simulink model "Main_Firmware"  (R2024b)
settings: Solver=FixedStepDiscrete  StartTime=0.0  StopTime=Inf  FixedStep=5e-06  RelTol=1e-3
values from neighbouring files (symbols this model uses):
  A_f = 1.24    [Minh_Inverter_Init.m]
  C_d = 0.7041    [Minh_Inverter_Init.m]
  C_rr = 0.02    [Minh_Inverter_Init.m]
  Current_max = min(InvCurr,mCurr)    [Minh_Inverter_Init.m]
  Encoder_Offset = -17.439*pi/180    (= -0.304367968255)    [Minh_Inverter_Init.m]
  EPWM_F = 200000    [Minh_Inverter_Init.m]
  g = 9.8    [Minh_Inverter_Init.m]
  J = mrot*r^2/k^2 + 0.0045    (= 0.8303048)    [Minh_Inverter_Init.m]
  k = 1    [Minh_Inverter_Init.m]
  lambda = 0.0375    [Minh_Inverter_Init.m]
  Ld = 0.1e-3    (= 0.0001)    [Minh_Inverter_Init.m]
  Lq = Ld    (= 0.0001)    [Minh_Inverter_Init.m]
  m = 1    [Minh_Inverter_Init.m]
  ppair = 4    [Minh_Inverter_Init.m]
  r = 0.4064/2    (= 0.2032)    [Minh_Inverter_Init.m]
  rho = 1.2    [Minh_Inverter_Init.m]
  Rs = (Rpp^2)/(Rpp*3)    (= 0.00433333333333)    [Minh_Inverter_Init.m]
  speed_max = rpm_max*2*pi/60    (= 523.598775598)    [Minh_Inverter_Init.m]
  Torque_max = Current_max*3*lambda*ppair/2    [Minh_Inverter_Init.m]
  Voltage_max = min(V_bat,mVolt)    [Minh_Inverter_Init.m]
undefined symbols (not defined in the file or in its folder): DiscIntNeverNeededParam, dspblkCoreblockFVToolHelper, gcbh, GPTRIP1SEL, TZ1
libraries: c2802xlib x4, c28004xlib x3, slpidlib x3, simulink x2, spsabctodq0Lib x2, spsdq0toabcLib x1
settings Model: SimulationMode=external  ExtModeTrigDuration=8  Creator=minhp  LastModifiedBy=minhp
settings OptimizationCC: DefaultUnderspecifiedDataType=single  EnhancedBackFolding=on  PassReuseOutputArgsAs=Individual arguments  MaxStackSize=1024  OptimizeBlockOrder=speed  DifferentSizesBufferReuse=on  OptimizationCustomize=off  EfficientTunableParamExpr=on
settings DebuggingCC: SingleTaskRateTransMsg=warning  ParameterTunabilityLossMsg=error
settings HardwareCC: ProdBitPerChar=16  ProdBitPerInt=16  ProdBitPerPointer=32  ProdBitPerSizeT=32  ProdBitPerPtrDiffT=32  ProdLargestAtomicInteger=Integer  ProdLargestAtomicFloat=None  ProdWordSize=16  ProdLongLongMode=on  ProdHWDeviceType=Texas Instruments->C2000  HardwareBoardFeatureSet=SoCBlockset
settings SFSimCC: MATLABDynamicMemAlloc=off
settings RTWCC: Description=Embedded Coder  SystemTargetFile=ert.tlc  HardwareBoard=TI Piccolo F280049C LaunchPad  TemplateMakefile=ert_default_tmf  Toolchain=Texas Instruments Code Composer Studio (C2000)  CodeProfilingSaveOptions=MetricsOnly
settings CodeAppCC: ForceParamTrailComments=on  IgnoreCustomStorageClasses=off  OperatorAnnotations=on  SimulinkDataObjDesc=on  SFDataObjDesc=on  InsertBlockDesc=on
settings ERTTargetCC: CodeReplacementLibrary=TI C28x  ExtModeTransport=4  ExtModeStaticAlloc=on  ExtModeAutomaticAllocSize=off  ExtModeStaticAllocSize=5000  ExtModeMexFile=ext_xcp  ExtModeIntrfLevel=Level2 - Open  InlinedParameterPlacement=Hierarchical  DynamicArrayContainerType=coder::array

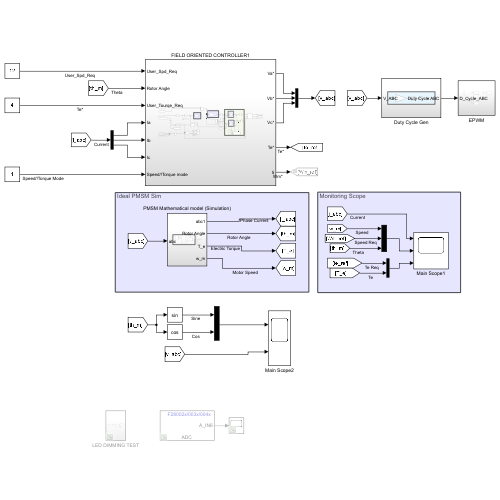
[thumbnail: Simulink's stored preview of the top-level diagram]
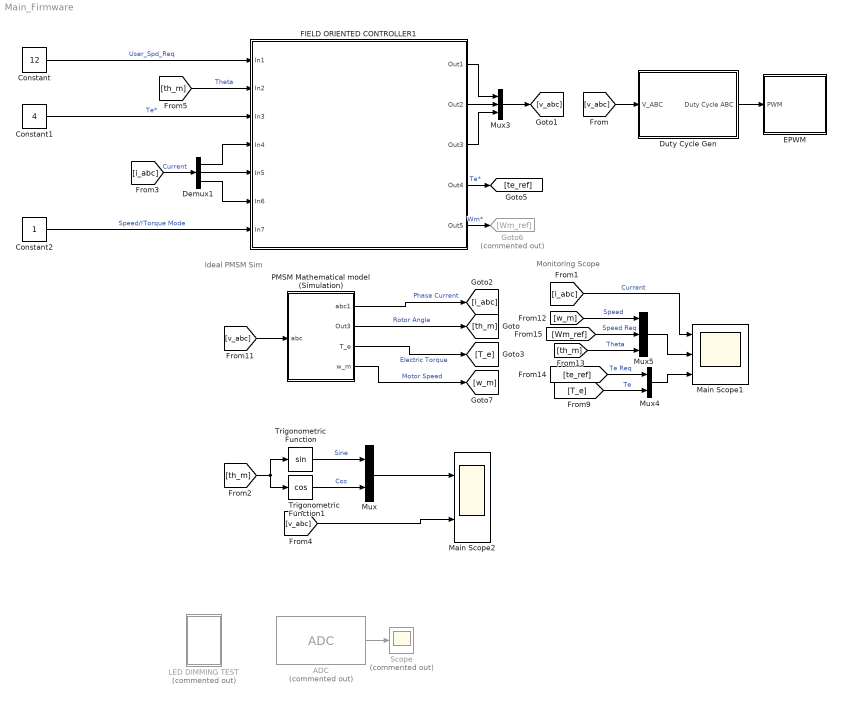
== system Main_Firmware ==
  note: Ideal PMSM Sim
  note: Monitoring Scope
  ADC : c2802xlib/ADC  Commented=on  blkParamProc=C2000_Type5  ADCModule=A  samplingMode=Single sample mode  ADCResolution=12-bit (Single-ended input)  useSOC1=SOC0  useSOC2=SOC0_SOC1  SOCAcquisitionWindow=8  SOCTriggerSource=Software  SOCInterruptTrigger=No ADCINT  Ts=0.001  dType=single  postInterrupt=off  interruptSel=ADCINT1  ADCINTContinuous=on  endma=off  chdma=1  conv1=ADCINA0  conv2=ADCINA0 and ADCINB0  conv1_Type4=ADCIN6  conv2_Type4=ADCIN0 and ADCIN1
      settings: LibrarySourceBlock=c28004xlib/ADC
  Constant : Constant  Value=12
  Constant1 : Constant  Value=4
  Constant2 : Constant
  Demux1 : Demux  Outputs=3
  Duty Cycle Gen : Subsystem
  EPWM : Subsystem
  FIELD ORIENTED CONTROLLER1 : Subsystem
  Goto6 : Goto  Commented=on  GotoTag=Wm_ref
  LED DIMMING TEST : Subsystem  Commented=on
  Main Scope1 : Scope  NumInputPorts=3
  Main Scope2 : Scope  NumInputPorts=2
  Mux : Mux  Inputs=2
  Mux3 : Mux  Inputs=3
  Mux4 : Mux  Inputs=2
  Mux5 : Mux  Inputs=3
  PMSM Mathematical model (Simulation) : Subsystem
  Scope : Scope  Commented=on
  Trigonometric Function : Trigonometry
  Trigonometric Function1 : Trigonometry  Operator=cos
  wires:
  ADC/1 -> Scope/1
  Duty Cycle Gen/1(Duty Cycle ABC) -> EPWM/1(PWM)
  PMSM Mathematical model (Simulation)/2(Out3) -> [th_m]  "Rotor Angle"
  PMSM Mathematical model (Simulation)/4(w_m) -> [w_m]  "Motor Speed"
  [v_abc] -> PMSM Mathematical model (Simulation)/1(abc)
  PMSM Mathematical model (Simulation)/1(abc1) -> [i_abc]  "Phase Current"
  PMSM Mathematical model (Simulation)/3(T_e) -> [T_e]  "Electric Torque"
  Constant1/1 -> FIELD ORIENTED CONTROLLER1/3(In3)  "Te*"
  FIELD ORIENTED CONTROLLER1/1(Out1) -> Mux3/1
  FIELD ORIENTED CONTROLLER1/4(Out4) -> [te_ref]  "Te*"
  FIELD ORIENTED CONTROLLER1/2(Out2) -> Mux3/2
  Mux3/1 -> [v_abc]
  FIELD ORIENTED CONTROLLER1/3(Out3) -> Mux3/3
  [i_abc] -> Demux1/1  "Current"
  [th_m] -> FIELD ORIENTED CONTROLLER1/2(In2)  "Theta"
  Demux1/2 -> FIELD ORIENTED CONTROLLER1/5(In5)
  Demux1/3 -> FIELD ORIENTED CONTROLLER1/6(In6)
  Constant2/1 -> FIELD ORIENTED CONTROLLER1/7(In7)  "Speed/!Torque Mode"
  Demux1/1 -> FIELD ORIENTED CONTROLLER1/4(In4)
  Constant/1 -> FIELD ORIENTED CONTROLLER1/1(In1)  "User_Spd_Req"
  FIELD ORIENTED CONTROLLER1/5(Out5) -> Goto6/1  "Wm*"
  [v_abc] -> Duty Cycle Gen/1(V_ABC)
  [th_m] -> Mux5/3  "Theta"
  [te_ref] -> Mux4/1  "Te Req"
  [T_e] -> Mux4/2  "Te"
  Mux5/1 -> Main Scope1/2
  [w_m] -> Mux5/1  "Speed"
  [Wm_ref] -> Mux5/2  "Speed Req"
  [i_abc] -> Main Scope1/1  "Current"
  Mux4/1 -> Main Scope1/3
  [th_m] -> Trigonometric Function1/1, Trigonometric Function/1
  Trigonometric Function1/1 -> Mux/2  "Cos"
  [v_abc] -> Main Scope2/2
  Trigonometric Function/1 -> Mux/1  "Sine"
  Mux/1 -> Main Scope2/1

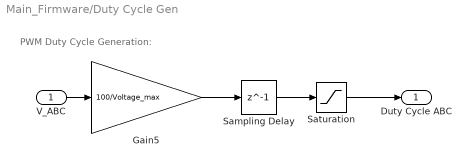
== system Main_Firmware/Duty Cycle Gen ==
  note: PWM Duty Cycle Generation:
  V_ABC : Inport
  Gain5 : Gain  Gain=100/Voltage_max
  Sampling Delay : Delay  DelayLength=1
  Saturation : Saturate  UpperLimit=100  LowerLimit=0
  Duty Cycle ABC : Outport
  wires:
  Sampling Delay/1 -> Saturation/1
  Gain5/1 -> Sampling Delay/1
  Saturation/1 -> Duty Cycle ABC/1
  V_ABC/1 -> Gain5/1

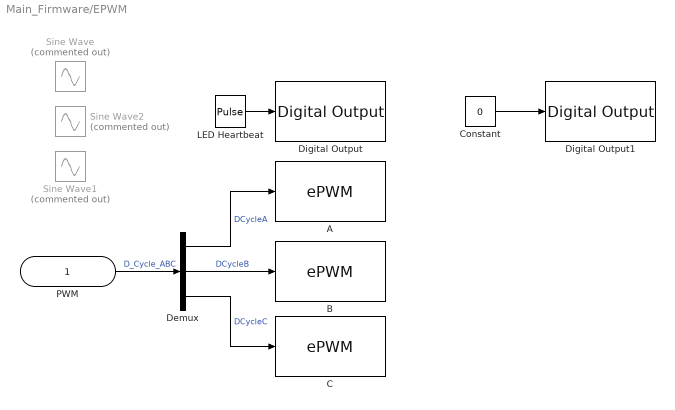
== system Main_Firmware/EPWM ==
  PWM : Inport
  A : c2802xlib/ePWM  PwmType=C2000_Type4  useModule=ePWM1  ePWMxLINKTBPRD=Not Linked  periodUnits=Seconds  timerSource=Specify via dialog  timerPeriod_clk=1/EPWM_F  timerPeriod_sec=1/EPWM_F  tbshadow=Counter equals to zero  countingMode=Up  phaseActiveEnable=Disable  phaseDirection=Count down after sync  phaseActive=0  synchronizationEnable=off  dcaevt1Sync=off  dcbevt1Sync=off  synchronizationOption=Disable  dcbevt1SyncOut=off  dcaevt1SyncOut=off  cmpdSyncOut=off  cmpcSyncOut=off  cmpbSyncOut=off  zeroSyncOut=off  swfSyncOut=off  perSynchronizationOption=Counter equals to period (CTR=PRD)  clockPrescale=1  HSclockPrescale=1  enswap=off  ePWMxAStatus=on  ePWMxAactionLogic1=Set  ePWMxAactionLogic2=Clear  ePWMxAactionLogic3=Clear  ePWMxAactionLogic4=Set  ePWMxAactionLogic5=Do nothing  ePWMxAactionLogic6=Do nothing  ePWMxACSFenable=off  ePWMxACSFvalue=Forcing disable  ePWMxASFreload=Zero  ePWMxBStatus=on  ePWMxBactionLogic1=Set  ePWMxBactionLogic2=Clear  ePWMxBactionLogic3=Clear  ePWMxBactionLogic4=Do nothing  ePWMxBactionLogic5=Do nothing  ePWMxBactionLogic6=Set  ePWMxBCSFenable=off  ePWMxBCSFvalue=Forcing disable  ePWMxBSFreload=Zero  ePWNxBOutWay=on  ePWMxLINKCMPA=Not Linked  CMPAUnits=Percentages  CMPASource=Input port  CMPAValue_per=0  CMPAValue_clk=0  enCMPAshadow=Counter equals to zero (CTR=Zero)  ePWMxLINKCMPB=Not Linked  CMPBUnits=Clock cycles  CMPBSource=Specify via dialog  CMPBValue_per=50  CMPBValue_clk=32000  enCMPBshadow=Counter equals to zero (CTR=Zero)  ePWMxLINKCMPC=Not Linked  CMPCUnits=Percentages  CMPCSource=Specify via dialog  CMPCValue_per=60  CMPCValue_clk=50  enCMPCshadow=Counter equals to zero (CTR=Zero)  ePWMxLINKCMPD=Not Linked  CMPDUnits=Clock cycles  CMPDSource=Specify via dialog  CMPDValue_per=50  CMPDValue_clk=32000  enCMPDshadow=Counter equals to zero (CTR=Zero)  enableDBePWMxA=off  enableDBePWMxB=off  enhalfcycle=off  DBpolarity=Active high (AH)  DBedgeDelay=Positive  DBSource_ePWMxA=ePWMxA  DBSource_ePWMxB=ePWMxA  DBPeriodUnits=Clock cycles  DBperiodSource=Specify via dialog  REDperiod=0  FEDperiod=0  REDperiod_sec=0  FEDperiod_sec=0  LoadModeDBRED=Immediate without using shadow  LoadModeDBFED=Immediate without using shadow  adcstartModuleA=off  adcrequestEventA=First event  adcstartEventA=Digital Compare Module A Event 1 start of conversion (DCAEVT1.soc)  adcstartEventA_type2=Counter equals to zero (CTR=Zero)  adcstartModuleB=off  adcrequestEventB=First event  adcstartEventB=Counter equals to zero (CTR=Zero)  adcstartEventB_type2=Counter equals to zero (CTR=Zero)  intEn=off  intPrd=First event  intSel=Counter equals to zero (CTR=Zero)  intSel_type2=Counter equals to zero (CTR=Zero)  hrpe=off  enHRPWM=off  HRPWM_LoadMode=Counter equals to period (CTR=PRD)  HRPWM_CTLMode=Duty or Period control mode  HRPWM_EDGMode=Both edge  hrpeb=off  enHRPWMB=off  HRPWM_LoadModeB=Counter equals to zero (CTR=ZERO)  HRPWM_CTLModeB=Duty or Period control mode  HRPWM_EDGModeB=Both edge  enHRDBRED=off  enHRDBFED=off  enSFO=on  enautoconv=on  chopperEnable=off  chopperFrequency=1  chopperFirstwidth=1  chopperDuty=12.5%  tripZonesource=Specify via dialog  tzselOSHT1=off  tzselOSHT2=off  tzselOSHT3=off  tzselOSHT4=off  tzselOSHT5=off  tzselOSHT6=off  tzselOSHDCAEV1=off  tzselOSHDCBEV1=off  tzselCBC1=off  tzselCBC2=off  tzselCBC3=off  tzselCBC4=off  tzselCBC5=off  tzselCBC6=off  tzselCBCDCAEV2=off  tzselCBCDCBEV2=off  enTzOstIntr=off  enTzCbcIntr=off  enTzDCAEVT1Intr=off  enTzDCAEVT2Intr=off  enTzDCBEVT1Intr=off  enTzDCBEVT2Intr=off  tzclrCBCLatch=Counter equals to zero (CTR=Zero)  ePWMxAforced=No action  ePWMxBforced=No action  DCAEVT1forced=No action  DCBEVT1forced=No action  DCAEVT2forced=No action  DCBEVT2forced=No action  dcah=Trip Zone 1 input (TZ1)  dcal=Trip Zone 2 input (TZ2)  dcbh=Trip Zone 1 input (TZ1)  dcbl=Trip Zone 2 input (TZ2)  dcah_type2=GPTRIP1SEL/(TZ1)  dcal_type2=GPTRIP1SEL/(TZ1)  dcbh_type2=GPTRIP1SEL/(TZ1)  dcbl_type2=GPTRIP1SEL/(TZ1)  gendcaevt1=Event disabled  gendcaevt2=Event disabled  gendcbevt1=Event disabled  gendcbevt2=Event disabled  dcaevt1src=DCAEVT1 with sync  dcaevt2src=DCAEVT2 with sync  dcbevt1src=DCBEVT1 with sync  dcbevt2src=DCBEVT2 with sync  pulsesel=Counter equals to zero (CTR=Zero)  blankinv=off  blankoffset=0  blankwidth=0  evsrcsel=Filtered version of DCAEVT1 (DCAEVT1FILT)  encape=off
      settings: LibrarySourceBlock=c28004xlib/ePWM
  B : c2802xlib/ePWM  PwmType=C2000_Type4  useModule=ePWM4  ePWMxLINKTBPRD=ePWM1  periodUnits=Seconds  timerSource=Specify via dialog  timerPeriod_clk=1/EPWM_F  timerPeriod_sec=1/EPWM_F  tbshadow=Counter equals to zero  countingMode=Up  phaseActiveEnable=Disable  phaseDirection=Count down after sync  phaseActive=0  synchronizationEnable=off  dcaevt1Sync=off  dcbevt1Sync=off  synchronizationOption=Disable  dcbevt1SyncOut=off  dcaevt1SyncOut=off  cmpdSyncOut=off  cmpcSyncOut=off  cmpbSyncOut=off  zeroSyncOut=off  swfSyncOut=off  perSynchronizationOption=Counter equals to period (CTR=PRD)  clockPrescale=1  HSclockPrescale=1  enswap=off  ePWMxAStatus=on  ePWMxAactionLogic1=Set  ePWMxAactionLogic2=Clear  ePWMxAactionLogic3=Clear  ePWMxAactionLogic4=Set  ePWMxAactionLogic5=Do nothing  ePWMxAactionLogic6=Do nothing  ePWMxACSFenable=off  ePWMxACSFvalue=Forcing disable  ePWMxASFreload=Zero  ePWMxBStatus=on  ePWMxBactionLogic1=Set  ePWMxBactionLogic2=Clear  ePWMxBactionLogic3=Clear  ePWMxBactionLogic4=Do nothing  ePWMxBactionLogic5=Do nothing  ePWMxBactionLogic6=Set  ePWMxBCSFenable=off  ePWMxBCSFvalue=Forcing disable  ePWMxBSFreload=Zero  ePWNxBOutWay=on  ePWMxLINKCMPA=Not Linked  CMPAUnits=Percentages  CMPASource=Input port  CMPAValue_per=0  CMPAValue_clk=0  enCMPAshadow=Counter equals to zero (CTR=Zero)  ePWMxLINKCMPB=Not Linked  CMPBUnits=Clock cycles  CMPBSource=Specify via dialog  CMPBValue_per=50  CMPBValue_clk=32000  enCMPBshadow=Counter equals to zero (CTR=Zero)  ePWMxLINKCMPC=Not Linked  CMPCUnits=Percentages  CMPCSource=Specify via dialog  CMPCValue_per=60  CMPCValue_clk=50  enCMPCshadow=Counter equals to zero (CTR=Zero)  ePWMxLINKCMPD=Not Linked  CMPDUnits=Clock cycles  CMPDSource=Specify via dialog  CMPDValue_per=50  CMPDValue_clk=32000  enCMPDshadow=Counter equals to zero (CTR=Zero)  enableDBePWMxA=off  enableDBePWMxB=off  enhalfcycle=off  DBpolarity=Active high (AH)  DBedgeDelay=Positive  DBSource_ePWMxA=ePWMxA  DBSource_ePWMxB=ePWMxA  DBPeriodUnits=Clock cycles  DBperiodSource=Specify via dialog  REDperiod=0  FEDperiod=0  REDperiod_sec=0  FEDperiod_sec=0  LoadModeDBRED=Immediate without using shadow  LoadModeDBFED=Immediate without using shadow  adcstartModuleA=off  adcrequestEventA=First event  adcstartEventA=Digital Compare Module A Event 1 start of conversion (DCAEVT1.soc)  adcstartEventA_type2=Counter equals to zero (CTR=Zero)  adcstartModuleB=off  adcrequestEventB=First event  adcstartEventB=Counter equals to zero (CTR=Zero)  adcstartEventB_type2=Counter equals to zero (CTR=Zero)  intEn=off  intPrd=First event  intSel=Counter equals to zero (CTR=Zero)  intSel_type2=Counter equals to zero (CTR=Zero)  hrpe=off  enHRPWM=off  HRPWM_LoadMode=Counter equals to period (CTR=PRD)  HRPWM_CTLMode=Duty or Period control mode  HRPWM_EDGMode=Both edge  hrpeb=off  enHRPWMB=off  HRPWM_LoadModeB=Counter equals to zero (CTR=ZERO)  HRPWM_CTLModeB=Duty or Period control mode  HRPWM_EDGModeB=Both edge  enHRDBRED=off  enHRDBFED=off  enSFO=on  enautoconv=on  chopperEnable=off  chopperFrequency=1  chopperFirstwidth=1  chopperDuty=12.5%  tripZonesource=Specify via dialog  tzselOSHT1=off  tzselOSHT2=off  tzselOSHT3=off  tzselOSHT4=off  tzselOSHT5=off  tzselOSHT6=off  tzselOSHDCAEV1=off  tzselOSHDCBEV1=off  tzselCBC1=off  tzselCBC2=off  tzselCBC3=off  tzselCBC4=off  tzselCBC5=off  tzselCBC6=off  tzselCBCDCAEV2=off  tzselCBCDCBEV2=off  enTzOstIntr=off  enTzCbcIntr=off  enTzDCAEVT1Intr=off  enTzDCAEVT2Intr=off  enTzDCBEVT1Intr=off  enTzDCBEVT2Intr=off  tzclrCBCLatch=Counter equals to zero (CTR=Zero)  ePWMxAforced=No action  ePWMxBforced=No action  DCAEVT1forced=No action  DCBEVT1forced=No action  DCAEVT2forced=No action  DCBEVT2forced=No action  dcah=Trip Zone 1 input (TZ1)  dcal=Trip Zone 2 input (TZ2)  dcbh=Trip Zone 1 input (TZ1)  dcbl=Trip Zone 2 input (TZ2)  dcah_type2=GPTRIP1SEL/(TZ1)  dcal_type2=GPTRIP1SEL/(TZ1)  dcbh_type2=GPTRIP1SEL/(TZ1)  dcbl_type2=GPTRIP1SEL/(TZ1)  gendcaevt1=Event disabled  gendcaevt2=Event disabled  gendcbevt1=Event disabled  gendcbevt2=Event disabled  dcaevt1src=DCAEVT1 with sync  dcaevt2src=DCAEVT2 with sync  dcbevt1src=DCBEVT1 with sync  dcbevt2src=DCBEVT2 with sync  pulsesel=Counter equals to zero (CTR=Zero)  blankinv=off  blankoffset=0  blankwidth=0  evsrcsel=Filtered version of DCAEVT1 (DCAEVT1FILT)  encape=off
      settings: LibrarySourceBlock=c28004xlib/ePWM
  C : c2802xlib/ePWM  PwmType=C2000_Type4  useModule=ePWM2  ePWMxLINKTBPRD=ePWM1  periodUnits=Seconds  timerSource=Specify via dialog  timerPeriod_clk=1/EPWM_F  timerPeriod_sec=1/EPWM_F  tbshadow=Counter equals to zero  countingMode=Up  phaseActiveEnable=Disable  phaseDirection=Count down after sync  phaseActive=0  synchronizationEnable=off  dcaevt1Sync=off  dcbevt1Sync=off  synchronizationOption=Disable  dcbevt1SyncOut=off  dcaevt1SyncOut=off  cmpdSyncOut=off  cmpcSyncOut=off  cmpbSyncOut=off  zeroSyncOut=off  swfSyncOut=off  perSynchronizationOption=Counter equals to period (CTR=PRD)  clockPrescale=1  HSclockPrescale=1  enswap=off  ePWMxAStatus=on  ePWMxAactionLogic1=Set  ePWMxAactionLogic2=Clear  ePWMxAactionLogic3=Clear  ePWMxAactionLogic4=Set  ePWMxAactionLogic5=Do nothing  ePWMxAactionLogic6=Do nothing  ePWMxACSFenable=off  ePWMxACSFvalue=Forcing disable  ePWMxASFreload=Zero  ePWMxBStatus=on  ePWMxBactionLogic1=Set  ePWMxBactionLogic2=Clear  ePWMxBactionLogic3=Clear  ePWMxBactionLogic4=Do nothing  ePWMxBactionLogic5=Do nothing  ePWMxBactionLogic6=Set  ePWMxBCSFenable=off  ePWMxBCSFvalue=Forcing disable  ePWMxBSFreload=Zero  ePWNxBOutWay=on  ePWMxLINKCMPA=Not Linked  CMPAUnits=Percentages  CMPASource=Input port  CMPAValue_per=0  CMPAValue_clk=0  enCMPAshadow=Counter equals to zero (CTR=Zero)  ePWMxLINKCMPB=Not Linked  CMPBUnits=Clock cycles  CMPBSource=Specify via dialog  CMPBValue_per=50  CMPBValue_clk=32000  enCMPBshadow=Counter equals to zero (CTR=Zero)  ePWMxLINKCMPC=Not Linked  CMPCUnits=Percentages  CMPCSource=Specify via dialog  CMPCValue_per=60  CMPCValue_clk=50  enCMPCshadow=Counter equals to zero (CTR=Zero)  ePWMxLINKCMPD=Not Linked  CMPDUnits=Clock cycles  CMPDSource=Specify via dialog  CMPDValue_per=50  CMPDValue_clk=32000  enCMPDshadow=Counter equals to zero (CTR=Zero)  enableDBePWMxA=off  enableDBePWMxB=off  enhalfcycle=off  DBpolarity=Active high (AH)  DBedgeDelay=Positive  DBSource_ePWMxA=ePWMxA  DBSource_ePWMxB=ePWMxA  DBPeriodUnits=Clock cycles  DBperiodSource=Specify via dialog  REDperiod=0  FEDperiod=0  REDperiod_sec=0  FEDperiod_sec=0  LoadModeDBRED=Immediate without using shadow  LoadModeDBFED=Immediate without using shadow  adcstartModuleA=off  adcrequestEventA=First event  adcstartEventA=Digital Compare Module A Event 1 start of conversion (DCAEVT1.soc)  adcstartEventA_type2=Counter equals to zero (CTR=Zero)  adcstartModuleB=off  adcrequestEventB=First event  adcstartEventB=Counter equals to zero (CTR=Zero)  adcstartEventB_type2=Counter equals to zero (CTR=Zero)  intEn=off  intPrd=First event  intSel=Counter equals to zero (CTR=Zero)  intSel_type2=Counter equals to zero (CTR=Zero)  hrpe=off  enHRPWM=off  HRPWM_LoadMode=Counter equals to period (CTR=PRD)  HRPWM_CTLMode=Duty or Period control mode  HRPWM_EDGMode=Both edge  hrpeb=off  enHRPWMB=off  HRPWM_LoadModeB=Counter equals to zero (CTR=ZERO)  HRPWM_CTLModeB=Duty or Period control mode  HRPWM_EDGModeB=Both edge  enHRDBRED=off  enHRDBFED=off  enSFO=on  enautoconv=on  chopperEnable=off  chopperFrequency=1  chopperFirstwidth=1  chopperDuty=12.5%  tripZonesource=Specify via dialog  tzselOSHT1=off  tzselOSHT2=off  tzselOSHT3=off  tzselOSHT4=off  tzselOSHT5=off  tzselOSHT6=off  tzselOSHDCAEV1=off  tzselOSHDCBEV1=off  tzselCBC1=off  tzselCBC2=off  tzselCBC3=off  tzselCBC4=off  tzselCBC5=off  tzselCBC6=off  tzselCBCDCAEV2=off  tzselCBCDCBEV2=off  enTzOstIntr=off  enTzCbcIntr=off  enTzDCAEVT1Intr=off  enTzDCAEVT2Intr=off  enTzDCBEVT1Intr=off  enTzDCBEVT2Intr=off  tzclrCBCLatch=Counter equals to zero (CTR=Zero)  ePWMxAforced=No action  ePWMxBforced=No action  DCAEVT1forced=No action  DCBEVT1forced=No action  DCAEVT2forced=No action  DCBEVT2forced=No action  dcah=Trip Zone 1 input (TZ1)  dcal=Trip Zone 2 input (TZ2)  dcbh=Trip Zone 1 input (TZ1)  dcbl=Trip Zone 2 input (TZ2)  dcah_type2=GPTRIP1SEL/(TZ1)  dcal_type2=GPTRIP1SEL/(TZ1)  dcbh_type2=GPTRIP1SEL/(TZ1)  dcbl_type2=GPTRIP1SEL/(TZ1)  gendcaevt1=Event disabled  gendcaevt2=Event disabled  gendcbevt1=Event disabled  gendcbevt2=Event disabled  dcaevt1src=DCAEVT1 with sync  dcaevt2src=DCAEVT2 with sync  dcbevt1src=DCBEVT1 with sync  dcbevt2src=DCBEVT2 with sync  pulsesel=Counter equals to zero (CTR=Zero)  blankinv=off  blankoffset=0  blankwidth=0  evsrcsel=Filtered version of DCAEVT1 (DCAEVT1FILT)  encape=off
      settings: LibrarySourceBlock=c28004xlib/ePWM
  Constant : Constant  Value=0
  Demux : Demux  Outputs=3
  Digital Output : c28004xlib/Digital Output  GPIO_Number=GPIO16~GPIO23  GPIO_Bit0=off  GPIO_BIT0_Toggle=off  GPIO_Bit1=off  GPIO_BIT1_Toggle=off  GPIO_Bit2=off  GPIO_BIT2_Toggle=off  GPIO_Bit3=off  GPIO_BIT3_Toggle=off  GPIO_Bit4=off  GPIO_BIT4_Toggle=off  GPIO_Bit5=off  GPIO_BIT5_Toggle=off  GPIO_Bit6=off  GPIO_BIT6_Toggle=off  GPIO_Bit7=on  GPIO_BIT7_Toggle=off
  Digital Output1 : c28004xlib/Digital Output  GPIO_Number=GPIO24~GPIO31  GPIO_Bit0=off  GPIO_BIT0_Toggle=off  GPIO_Bit1=off  GPIO_BIT1_Toggle=off  GPIO_Bit2=off  GPIO_BIT2_Toggle=off  GPIO_Bit3=off  GPIO_BIT3_Toggle=off  GPIO_Bit4=off  GPIO_BIT4_Toggle=off  GPIO_Bit5=off  GPIO_BIT5_Toggle=off  GPIO_Bit6=off  GPIO_BIT6_Toggle=off  GPIO_Bit7=on  GPIO_BIT7_Toggle=off
  LED Heartbeat : DiscretePulseGenerator  PulseType=Time based  Period=1  PulseWidth=50
  Sine Wave : Sin  Commented=on  Amplitude=50  Bias=50  Frequency=0.1*2*pi  SampleTime=0
  Sine Wave1 : Sin  Commented=on  Amplitude=50  Bias=50  Frequency=0.1*2*pi  Phase=-2*pi/3  SampleTime=0
  Sine Wave2 : Sin  Commented=on  Amplitude=50  Bias=50  Frequency=0.1*2*pi  Phase=2*pi/3  SampleTime=0
  wires:
  LED Heartbeat/1 -> Digital Output/1
  Constant/1 -> Digital Output1/1
  Demux/2 -> B/1  "DCycleB"
  Demux/3 -> C/1  "DCycleC"
  PWM/1 -> Demux/1  "D_Cycle_ABC"
  Demux/1 -> A/1  "DCycleA"

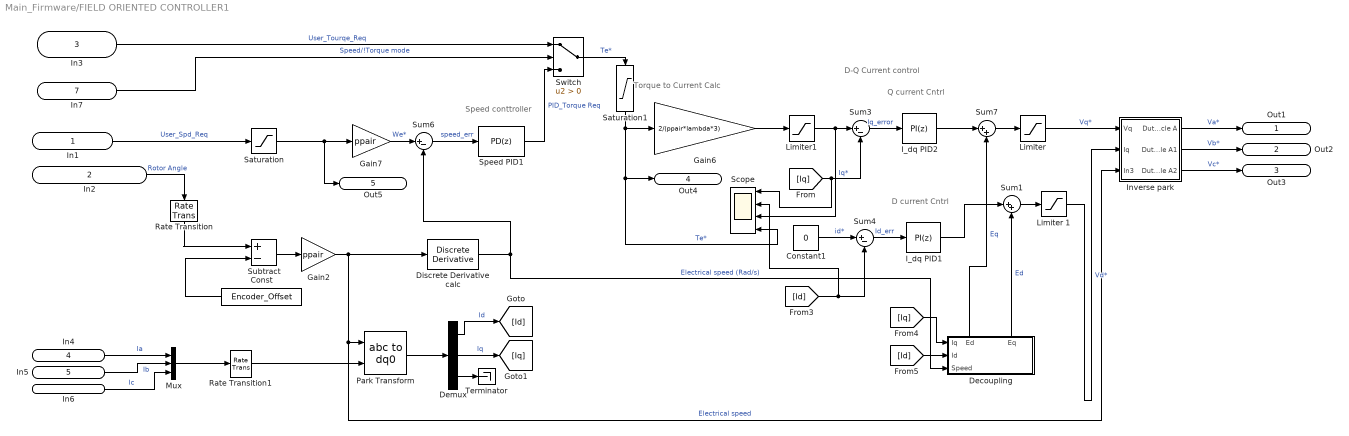
== system Main_Firmware/FIELD ORIENTED CONTROLLER1 ==
  note: Torque to Current Calc
  note: Speed conttroller
  note: D current
      | Cntrl
  note: D-Q Current control
  note: Q current
      | Cntrl
  In1 : Inport
  In2 : Inport  Port=2
  In3 : Inport  Port=3
  In4 : Inport  Port=4
  In5 : Inport  Port=5
  In6 : Inport  Port=6
  In7 : Inport  Port=7
  Const : Constant  Value=Encoder_Offset
  Constant1 : Constant  Value=0
  Decoupling : Subsystem
      settings: PortSchema="{\"entries\":[{\"content\":{\"sides\":[{\"content\":{\"connectorIds\":[\"In1\",\"In2\",\"In3\"]},\"type\":\"ConnectorPlacement.EquallySpacedRectSide\",\"uuid\":\"5f512ccb-8595-4499-a419-e995908cd1f5\"},{\"content\":{\"side\":\"RIGHT\"},\"type\":\"ConnectorPlacement.EquallySpacedRectSide\",\"uuid\":\"2a1de219-597a-4818-9587-d28590d7f25d\"},{\"content\":{\"connectorIds\":[\"Out1\",\"Out2\"],\"side\":\"TOP\"},\"type\":\"ConnectorPlacement.EquallySpacedRectSide\",\"uuid\":\"87b053a8-3806-4156-bae7-a97f33c02d51\"}]},\"type\":\"ConnectorPlacement.EquallySpacedConnector\",\"uuid\":\"5d9f8914-d3c5-4fbe-94a4-f1d2e0d8a5f7\"}],\"packageUris\":[\"http://schema.mathworks.com/mf0/Connector/R2020b\"],\"version\":\"1.0\"}"
  Demux : Demux  Outputs=3
  Discrete Derivative calc : simulink/Discrete/Discrete Derivative  gainval=1.0  ICPrevScaledInput=0.0  OutMin=[]  OutMax=[]  OutDataType=fixdt(1, 16)  OutScaling=2^-10  DoSatur=off
  Gain2 : Gain  Gain=ppair
  Gain6 : Gain  Gain=2/(ppair*lambda*3)
  Gain7 : Gain  Gain=ppair
  I_dq PID1 : slpidlib/PID Controller  Controller=PI  Form=Parallel  TimeDomain=Discrete-time  UseExternalTs=off  SampleTime=-1  IntegratorMethod=Forward Euler  FilterMethod=Forward Euler  ControllerParametersSource=internal  P=0.216674080570424  I=8.23559930371868  UseKiTs=off  D=2.81416629288768e-05  UseExternalDerivativeSource=off  N=4271.19819316481  UseFilter=on  TunerSelectOption=Transfer Function Based (PID Tuner App)  InitialConditionSource=internal  InitialConditionForIntegrator=0  InitialConditionForFilter=0  DifferentiatorICPrevScaledInput=0  ExternalReset=none  TrackingMode=off  Kt=1  LimitOutput=on  SatLimitsSource=internal  UpperSaturationLimit=Voltage_max  LowerSaturationLimit=-Voltage_max  LinearizeAsGain=off  AntiWindupMode=none  Kb=1  LimitIntegrator=on  UpperIntegratorSaturationLimit=Voltage_max  LowerIntegratorSaturationLimit=-Voltage_max  POutMin=[]  POutMax=[]  IOutMin=[]  IOutMax=[]  DOutMin=[]  DOutMax=[]  NOutMin=[]  NOutMax=[]  SumOutMin=[]  SumOutMax=[]  SaturationOutMin=[]  SaturationOutMax=[]  PParamMin=[]  PParamMax=[]  IParamMin=[]  IParamMax=[]  DParamMin=[]  DParamMax=[]  NParamMin=[]  NParamMax=[]  KbParamMin=[]  KbParamMax=[]  KtParamMin=[]  KtParamMax=[]  KbOutMin=[]  KbOutMax=[]  KtOutMin=[]  KtOutMax=[]  IntegratorOutMin=[]  IntegratorOutMax=[]  FilterOutMin=[]  FilterOutMax=[]  SumI1OutMin=[]  SumI1OutMax=[]  SumI2OutMin=[]  SumI2OutMax=[]  SumI3OutMin=[]  SumI3OutMax=[]  SumI4OutMin=[]  SumI4OutMax=[]  SumDOutMin=[]  SumDOutMax=[]  DifferentiatorOutMin=[]  DifferentiatorOutMax=[]  FilterDiffOutCoefMin=[]  FilterDiffOutCoefMax=[]  ReciprocalOutMin=[]  ReciprocalOutMax=[]  SumDenOutMin=[]  SumDenOutMax=[]  SumNumOutMin=[]  SumNumOutMax=[]  DivideOutMin=[]  DivideOutMax=[]  UdiffTsProdOutMin=[]  UdiffTsProdOutMax=[]  NTsProdOutMin=[]  NTsProdOutMax=[]  UintegralTsProdOutMin=[]  UintegralTsProdOutMax=[]  UngainTsProdOutMin=[]  UngainTsProdOutMax=[]  ClampingZeroOutDataTypeStr=Inherit: Inherit via back propagation  ClampingZeroOutMin=[]  ClampingZeroOutMax=[]  FilterDenConstantOutDataTypeStr=Inherit: Inherit via back propagation  FilterDenConstantOutMin=[]  FilterDenConstantOutMax=[]  PCopyOutDataTypeStr=Inherit: Inherit via back propagation  PCopyOutMin=[]  PCopyOutMax=[]  NCopyOutDataTypeStr=Inherit: Inherit via back propagation  NCopyOutMin=[]  NCopyOutMax=[]  IntegratorContinuousStateAttributes=''  IntegratorStateMustResolveToSignalObject=off  IntegratorRTWStateStorageClass=Auto  FilterContinuousStateAttributes=''  FilterStateMustResolveToSignalObject=off  FilterRTWStateStorageClass=Auto  ParallelPVariant=InternalParameters  IdealPVariant=Disabled  IVariant=InternalParameters  DVariant=Disabled  IntegratorVariant=Discrete  SatVariant=Enabled  AWVariant=Passthrough  PCopyVariant=Disabled  TRVariant=Disabled  FdbkBlocksVariant=Forward  IdealPFdbkVariant=Disabled  SatFdbkVariant=Disabled  DerivativeFilterVariant=Disabled  NVariant=Disabled  NCopyVariant=Disabled_SignalSpec  FilterICVariant=Disabled  IntegratorICVariant=InternalICs  ExternalResetVariant=Disabled  TRSumVariant=Passthrough  SumFdbkVariant=Disabled  SumVariant=Sum_PI  TsampFilterVariant=InternalTs  TsampNgainVariant=Passthrough  TsampIntegralVariant=Disabled_SignalSpec  ExternalSaturationOutDataTypeStr=Inherit: Same as second input  DerivativeSourceVariant=Disabled  PreIntVariant=InternalPreInt
  I_dq PID2 : slpidlib/PID Controller  Controller=PI  Form=Parallel  TimeDomain=Discrete-time  UseExternalTs=off  SampleTime=-1  IntegratorMethod=Forward Euler  FilterMethod=Forward Euler  ControllerParametersSource=internal  P=0.216674080570424  I=8.23559930371868  UseKiTs=off  D=2.81416629288768e-05  UseExternalDerivativeSource=off  N=4271.19819316481  UseFilter=on  TunerSelectOption=Transfer Function Based (PID Tuner App)  InitialConditionSource=internal  InitialConditionForIntegrator=0  InitialConditionForFilter=0  DifferentiatorICPrevScaledInput=0  ExternalReset=none  TrackingMode=off  Kt=1  LimitOutput=on  SatLimitsSource=internal  UpperSaturationLimit=Voltage_max  LowerSaturationLimit=-Voltage_max  LinearizeAsGain=off  AntiWindupMode=none  Kb=1  LimitIntegrator=on  UpperIntegratorSaturationLimit=Voltage_max  LowerIntegratorSaturationLimit=-Voltage_max  POutMin=[]  POutMax=[]  IOutMin=[]  IOutMax=[]  DOutMin=[]  DOutMax=[]  NOutMin=[]  NOutMax=[]  SumOutMin=[]  SumOutMax=[]  SaturationOutMin=[]  SaturationOutMax=[]  PParamMin=[]  PParamMax=[]  IParamMin=[]  IParamMax=[]  DParamMin=[]  DParamMax=[]  NParamMin=[]  NParamMax=[]  KbParamMin=[]  KbParamMax=[]  KtParamMin=[]  KtParamMax=[]  KbOutMin=[]  KbOutMax=[]  KtOutMin=[]  KtOutMax=[]  IntegratorOutMin=[]  IntegratorOutMax=[]  FilterOutMin=[]  FilterOutMax=[]  SumI1OutMin=[]  SumI1OutMax=[]  SumI2OutMin=[]  SumI2OutMax=[]  SumI3OutMin=[]  SumI3OutMax=[]  SumI4OutMin=[]  SumI4OutMax=[]  SumDOutMin=[]  SumDOutMax=[]  DifferentiatorOutMin=[]  DifferentiatorOutMax=[]  FilterDiffOutCoefMin=[]  FilterDiffOutCoefMax=[]  ReciprocalOutMin=[]  ReciprocalOutMax=[]  SumDenOutMin=[]  SumDenOutMax=[]  SumNumOutMin=[]  SumNumOutMax=[]  DivideOutMin=[]  DivideOutMax=[]  UdiffTsProdOutMin=[]  UdiffTsProdOutMax=[]  NTsProdOutMin=[]  NTsProdOutMax=[]  UintegralTsProdOutMin=[]  UintegralTsProdOutMax=[]  UngainTsProdOutMin=[]  UngainTsProdOutMax=[]  ClampingZeroOutDataTypeStr=Inherit: Inherit via back propagation  ClampingZeroOutMin=[]  ClampingZeroOutMax=[]  FilterDenConstantOutDataTypeStr=Inherit: Inherit via back propagation  FilterDenConstantOutMin=[]  FilterDenConstantOutMax=[]  PCopyOutDataTypeStr=Inherit: Inherit via back propagation  PCopyOutMin=[]  PCopyOutMax=[]  NCopyOutDataTypeStr=Inherit: Inherit via back propagation  NCopyOutMin=[]  NCopyOutMax=[]  IntegratorContinuousStateAttributes=''  IntegratorStateMustResolveToSignalObject=off  IntegratorRTWStateStorageClass=Auto  FilterContinuousStateAttributes=''  FilterStateMustResolveToSignalObject=off  FilterRTWStateStorageClass=Auto  ParallelPVariant=InternalParameters  IdealPVariant=Disabled  IVariant=InternalParameters  DVariant=Disabled  IntegratorVariant=Discrete  SatVariant=Enabled  AWVariant=Passthrough  PCopyVariant=Disabled  TRVariant=Disabled  FdbkBlocksVariant=Forward  IdealPFdbkVariant=Disabled  SatFdbkVariant=Disabled  DerivativeFilterVariant=Disabled  NVariant=Disabled  NCopyVariant=Disabled_SignalSpec  FilterICVariant=Disabled  IntegratorICVariant=InternalICs  ExternalResetVariant=Disabled  TRSumVariant=Passthrough  SumFdbkVariant=Disabled  SumVariant=Sum_PI  TsampFilterVariant=InternalTs  TsampNgainVariant=Passthrough  TsampIntegralVariant=Disabled_SignalSpec  ExternalSaturationOutDataTypeStr=Inherit: Same as second input  DerivativeSourceVariant=Disabled  PreIntVariant=InternalPreInt
  Inverse park : Subsystem
  Limiter : Saturate  UpperLimit=Voltage_max  LowerLimit=0  LinearizeAsGain=off
  Limiter 1 : Saturate  UpperLimit=Voltage_max  LowerLimit=0  LinearizeAsGain=off
  Limiter1 : Saturate  UpperLimit=Current_max  LowerLimit=-Current_max  LinearizeAsGain=off
  Mux : Mux  Inputs=3
  Park Transform : spsabctodq0Lib/abc to dq0  Alignment=Aligned with phase A axis
  Rate Transition : RateTransition  OutPortSampleTime=1/EPWM_F
  Rate Transition1 : RateTransition  OutPortSampleTime=1/EPWM_F
  Saturation : Saturate  UpperLimit=speed_max  LowerLimit=-speed_max
  Saturation1 : Saturate  UpperLimit=Torque_max  LowerLimit=-Torque_max
  Scope : Scope  NumInputPorts=4
  Speed PID1 : slpidlib/PID Controller  Controller=PD  Form=Parallel  TimeDomain=Discrete-time  UseExternalTs=off  SampleTime=-1  IntegratorMethod=Forward Euler  FilterMethod=Forward Euler  ControllerParametersSource=internal  P=20.6545195236646  I=640.266262711417  UseKiTs=off  D=0.00205517598679868  UseExternalDerivativeSource=off  N=100.498329175013  UseFilter=on  TunerSelectOption=Transfer Function Based (PID Tuner App)  InitialConditionSource=internal  InitialConditionForIntegrator=0  InitialConditionForFilter=0  DifferentiatorICPrevScaledInput=0  ExternalReset=none  TrackingMode=off  Kt=1  LimitOutput=on  SatLimitsSource=internal  UpperSaturationLimit=Torque_max  LowerSaturationLimit=-Torque_max  LinearizeAsGain=off  AntiWindupMode=none  Kb=1  LimitIntegrator=on  UpperIntegratorSaturationLimit=Torque_max  LowerIntegratorSaturationLimit=-Torque_max  RndMeth=Nearest  POutMin=[]  POutMax=[]  IOutMin=[]  IOutMax=[]  DOutMin=[]  DOutMax=[]  NOutMin=[]  NOutMax=[]  SumOutMin=[]  SumOutMax=[]  SaturationOutMin=[]  SaturationOutMax=[]  PParamMin=[]  PParamMax=[]  IParamMin=[]  IParamMax=[]  DParamMin=[]  DParamMax=[]  NParamMin=[]  NParamMax=[]  KbParamMin=[]  KbParamMax=[]  KtParamMin=[]  KtParamMax=[]  KbOutMin=[]  KbOutMax=[]  KtOutMin=[]  KtOutMax=[]  IntegratorOutMin=[]  IntegratorOutMax=[]  FilterOutMin=[]  FilterOutMax=[]  SumI1OutMin=[]  SumI1OutMax=[]  SumI2OutMin=[]  SumI2OutMax=[]  SumI3OutMin=[]  SumI3OutMax=[]  SumI4OutMin=[]  SumI4OutMax=[]  SumDOutMin=[]  SumDOutMax=[]  DifferentiatorOutMin=[]  DifferentiatorOutMax=[]  FilterDiffOutCoefMin=[]  FilterDiffOutCoefMax=[]  ReciprocalOutMin=[]  ReciprocalOutMax=[]  SumDenOutMin=[]  SumDenOutMax=[]  SumNumOutMin=[]  SumNumOutMax=[]  DivideOutMin=[]  DivideOutMax=[]  UdiffTsProdOutMin=[]  UdiffTsProdOutMax=[]  NTsProdOutMin=[]  NTsProdOutMax=[]  UintegralTsProdOutMin=[]  UintegralTsProdOutMax=[]  UngainTsProdOutMin=[]  UngainTsProdOutMax=[]  ClampingZeroOutDataTypeStr=Inherit: Inherit via back propagation  ClampingZeroOutMin=[]  ClampingZeroOutMax=[]  FilterDenConstantOutDataTypeStr=Inherit: Inherit via back propagation  FilterDenConstantOutMin=[]  FilterDenConstantOutMax=[]  PCopyOutDataTypeStr=Inherit: Inherit via back propagation  PCopyOutMin=[]  PCopyOutMax=[]  NCopyOutDataTypeStr=Inherit: Inherit via back propagation  NCopyOutMin=[]  NCopyOutMax=[]  IntegratorContinuousStateAttributes=''  IntegratorStateMustResolveToSignalObject=off  IntegratorRTWStateStorageClass=Auto  FilterContinuousStateAttributes=''  FilterStateMustResolveToSignalObject=off  FilterRTWStateStorageClass=Auto  ParallelPVariant=InternalParameters  IdealPVariant=Disabled  IVariant=Disabled  DVariant=InternalParameters  IntegratorVariant=Disabled  SatVariant=Enabled  AWVariant=Disabled  PCopyVariant=Disabled  TRVariant=Disabled  FdbkBlocksVariant=Forward  IdealPFdbkVariant=Disabled  SatFdbkVariant=Disabled  DerivativeFilterVariant=ForwardEulerFilter  NVariant=InternalParameters  NCopyVariant=Disabled  FilterICVariant=InternalICsFilter  IntegratorICVariant=Disabled  ExternalResetVariant=Disabled  TRSumVariant=Passthrough  SumFdbkVariant=Disabled  SumVariant=Sum_PD  TsampFilterVariant=InternalTs  TsampNgainVariant=Passthrough  TsampIntegralVariant=Disabled_SignalSpec  ExternalSaturationOutDataTypeStr=Inherit: Same as second input  DerivativeSourceVariant=ErrorSignal  PreIntVariant=InternalPreInt
  Subtract : Sum  Inputs=+-
  Sum1 : Sum  Inputs=|++
  Sum3 : Sum  Inputs=|+-
  Sum4 : Sum  Inputs=|+-
  Sum6 : Sum  Inputs=|+-
  Sum7 : Sum  Inputs=|++
  Switch : Switch  Criteria=u2 > Threshold  SaturateOnIntegerOverflow=off  InputSameDT=off
  Terminator : Terminator
  Out1 : Outport
  Out2 : Outport  Port=2
  Out3 : Outport  Port=3
  Out4 : Outport  Port=4
  Out5 : Outport  Port=5
  wires:
  In5/1 -> Mux/2  "Ib"
  In6/1 -> Mux/3  "Ic"
  Discrete Derivative calc/1 -> Decoupling/3(Speed), Sum6/2  "Electrical speed (Rad/s)"
  I_dq PID1/1 -> Sum1/1
  [Id] -> Scope/2, Sum4/2
  Demux/2 -> [Iq]  "Iq"
  Inverse park/1(Duty Cycle A) -> Out1/1  "Va*"
  I_dq PID2/1 -> Sum7/1
  Inverse park/3(Duty Cycle A2) -> Out3/1  "Vc*"
  [Iq] -> Scope/1, Sum3/2
  Saturation1/1 -> Scope/4, Out4/1, Gain6/1  "Te*"
  Demux/1 -> [Id]  "Id"
  [Iq] -> Decoupling/1(Iq)
  Demux/3 -> Terminator/1
  Sum3/1 -> I_dq PID2/1  "Iq_error"
  Decoupling/2(Eq) -> Sum1/2  "Ed"
  Sum7/1 -> Limiter/1
  Limiter 1/1 -> Inverse park/2(Iq)  "Vd*"
  Decoupling/1(Ed) -> Sum7/2  "Eq"
  In1/1 -> Saturation/1  "User_Spd_Req"
  Inverse park/2(Duty Cycle A1) -> Out2/1  "Vb*"
  Sum4/1 -> I_dq PID1/1  "Id_err"
  Sum1/1 -> Limiter 1/1
  Sum6/1 -> Speed PID1/1  "speed_err"
  Constant1/1 -> Sum4/1  "id*"
  Speed PID1/1 -> Switch/3  "PID_Torque Req"
  [Id] -> Decoupling/2(Id)
  In4/1 -> Mux/1  "Ia"
  Limiter/1 -> Inverse park/1(Vq)  "Vq*"
  Mux/1 -> Rate Transition1/1
  Gain6/1 -> Limiter1/1
  In3/1 -> Switch/1  "User_Tourqe_Req"
  Park Transform/1 -> Demux/1
  In2/1 -> Rate Transition/1  "Rotor Angle"
  In7/1 -> Switch/2  "Speed/!Torque mode"
  Limiter1/1 -> Scope/3, Sum3/1  "Iq*"
  Gain7/1 -> Sum6/1  "We*"
  Gain2/1 -> Discrete Derivative calc/1, Inverse park/3(In3), Park Transform/2  "Electrical speed"
  Const/1 -> Subtract/2
  Subtract/1 -> Gain2/1
  Rate Transition/1 -> Subtract/1
  Rate Transition1/1 -> Park Transform/1
  Switch/1 -> Saturation1/1  "Te*"
  Saturation/1 -> Out5/1, Gain7/1

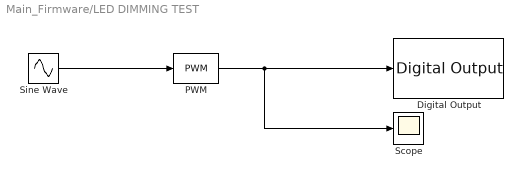
== system Main_Firmware/LED DIMMING TEST ==
  Digital Output : c28004xlib/Digital Output  GPIO_Number=GPIO16~GPIO23  GPIO_Bit0=off  GPIO_BIT0_Toggle=off  GPIO_Bit1=off  GPIO_BIT1_Toggle=off  GPIO_Bit2=off  GPIO_BIT2_Toggle=off  GPIO_Bit3=off  GPIO_BIT3_Toggle=off  GPIO_Bit4=off  GPIO_BIT4_Toggle=off  GPIO_Bit5=off  GPIO_BIT5_Toggle=off  GPIO_Bit6=off  GPIO_BIT6_Toggle=off  GPIO_Bit7=on  GPIO_BIT7_Toggle=off
  PWM : simulink/Discontinuities/PWM  DisableCoverage=on  Period=5e-2  InitialDelay=0.01  DisallowZeroDutyCycle=off  RunAtFixedTimeIntervals=on  SampleTime=0.001
  Scope : Scope
  Sine Wave : Sin  Amplitude=0.5  Bias=0.5  Frequency=2*2*pi  SampleTime=0
  wires:
  PWM/1 -> Scope/1, Digital Output/1
  Sine Wave/1 -> PWM/1

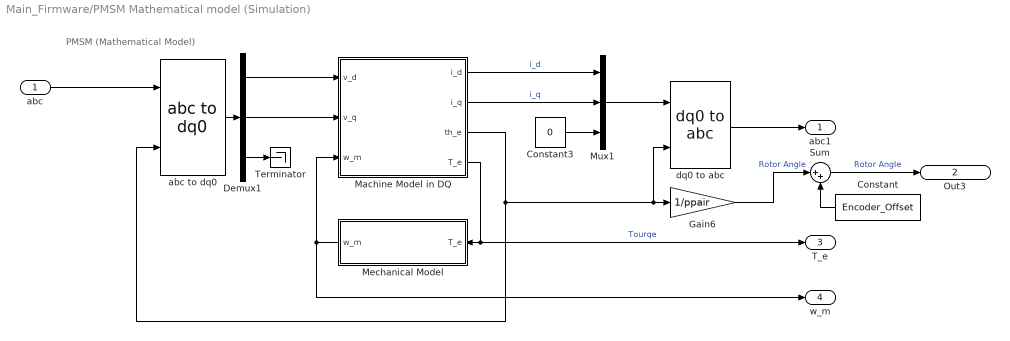
== system Main_Firmware/PMSM Mathematical model (Simulation) ==
  note: PMSM (Mathematical Model)
  abc : Inport
  Constant : Constant  Value=Encoder_Offset
  Constant3 : Constant  Value=0
  Demux1 : Demux  Outputs=3
  Gain6 : Gain  Gain=1/ppair
  Machine Model in DQ : Subsystem
  Mechanical Model : Subsystem
  Mux1 : Mux  Inputs=3
  Sum : Sum  Inputs=|++
  Terminator : Terminator
  abc to dq0 : spsabctodq0Lib/abc to dq0  Alignment=Aligned with phase A axis
  dq0 to abc : spsdq0toabcLib/dq0 to abc  Alignment=Aligned with phase A axis
  abc1 : Outport
  Out3 : Outport  Port=2
  T_e : Outport  Port=3
  w_m : Outport  Port=4
  wires:
  Demux1/2 -> Machine Model in DQ/2(v_q)
  Machine Model in DQ/3(th_e) -> abc to dq0/2, dq0 to abc/2, Gain6/1
  Demux1/1 -> Machine Model in DQ/1(v_d)
  Mux1/1 -> dq0 to abc/1
  Mechanical Model/1(w_m) -> w_m/1, Machine Model in DQ/3(w_m)
  Machine Model in DQ/4(T_e) -> T_e/1, Mechanical Model/1(T_e)  "Tourqe"
  Constant3/1 -> Mux1/3
  Demux1/3 -> Terminator/1
  Machine Model in DQ/1(i_d) -> Mux1/1  "i_d"
  Machine Model in DQ/2(i_q) -> Mux1/2  "i_q"
  abc to dq0/1 -> Demux1/1
  dq0 to abc/1 -> abc1/1
  abc/1 -> abc to dq0/1
  Gain6/1 -> Sum/1  "Rotor Angle"
  Sum/1 -> Out3/1  "Rotor Angle"
  Constant/1 -> Sum/2

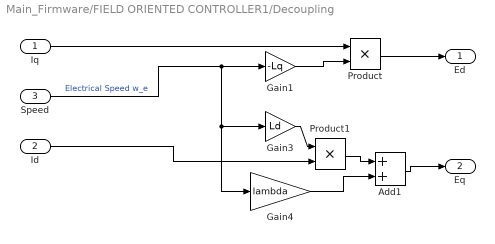
== system Main_Firmware/FIELD ORIENTED CONTROLLER1/Decoupling ==
  Iq : Inport
  Id : Inport  Port=2
  Speed : Inport  Port=3
  Add1 : Sum
  Gain1 : Gain  Gain=-Lq
  Gain3 : Gain  Gain=Ld
  Gain4 : Gain  Gain=lambda
  Product : Product
  Product1 : Product
  Ed : Outport
  Eq : Outport  Port=2
  wires:
  Product/1 -> Ed/1
  Gain3/1 -> Product1/1
  Product1/1 -> Add1/1
  Gain4/1 -> Add1/2
  Add1/1 -> Eq/1
  Speed/1 -> Gain4/1, Gain3/1, Gain1/1  "Electrical Speed w_e"
  Iq/1 -> Product/1
  Gain1/1 -> Product/2
  Id/1 -> Product1/2

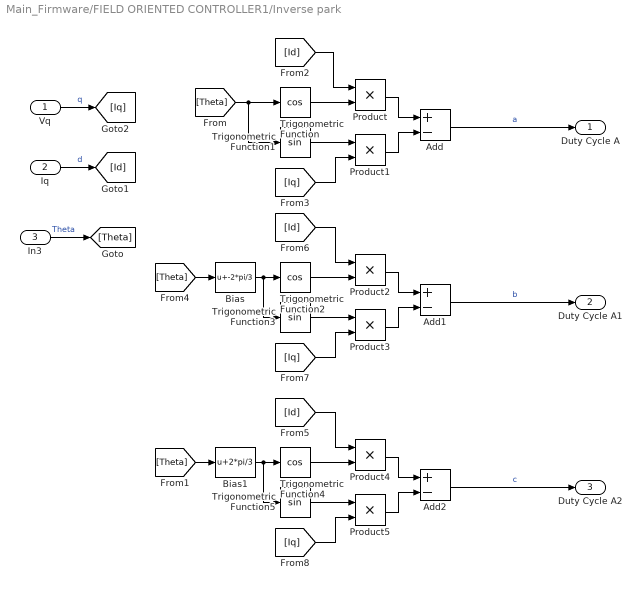
== system Main_Firmware/FIELD ORIENTED CONTROLLER1/Inverse park ==
  Vq : Inport
  Iq : Inport  Port=2
  In3 : Inport  Port=3
  Add : Sum  Inputs=+-
  Add1 : Sum  Inputs=+-
  Add2 : Sum  Inputs=+-
  Bias : Bias  Bias=-2*pi/3  SaturateOnIntegerOverflow=off
  Bias1 : Bias  Bias=2*pi/3  SaturateOnIntegerOverflow=off
  Product{,1..5} (6 alike) : Product
  Trigonometric Function : Trigonometry  Operator=cos
  Trigonometric Function1 : Trigonometry
  Trigonometric Function2 : Trigonometry  Operator=cos
  Trigonometric Function3 : Trigonometry
  Trigonometric Function4 : Trigonometry  Operator=cos
  Trigonometric Function5 : Trigonometry
  Duty Cycle A : Outport
  Duty Cycle A1 : Outport  Port=2
  Duty Cycle A2 : Outport  Port=3
  wires:
  Iq/1 -> [Id]  "d"
  Vq/1 -> [Iq]  "q"
  Add/1 -> Duty Cycle A/1  "a"
  Add1/1 -> Duty Cycle A1/1  "b"
  In3/1 -> [Theta]  "Theta"
  [Theta] -> Trigonometric Function1/1, Trigonometric Function/1
  [Iq] -> Product1/2
  Trigonometric Function/1 -> Product/2
  [Id] -> Product/1
  Trigonometric Function1/1 -> Product1/1
  Product/1 -> Add/1
  Product1/1 -> Add/2
  Product3/1 -> Add1/2
  [Theta] -> Bias/1
  [Id] -> Product2/1
  Product2/1 -> Add1/1
  Trigonometric Function3/1 -> Product3/1
  [Iq] -> Product3/2
  Trigonometric Function2/1 -> Product2/2
  Bias/1 -> Trigonometric Function3/1, Trigonometric Function2/1
  Trigonometric Function4/1 -> Product4/2
  [Id] -> Product4/1
  [Theta] -> Bias1/1
  [Iq] -> Product5/2
  Add2/1 -> Duty Cycle A2/1  "c"
  Product5/1 -> Add2/2
  Trigonometric Function5/1 -> Product5/1
  Product4/1 -> Add2/1
  Bias1/1 -> Trigonometric Function5/1, Trigonometric Function4/1

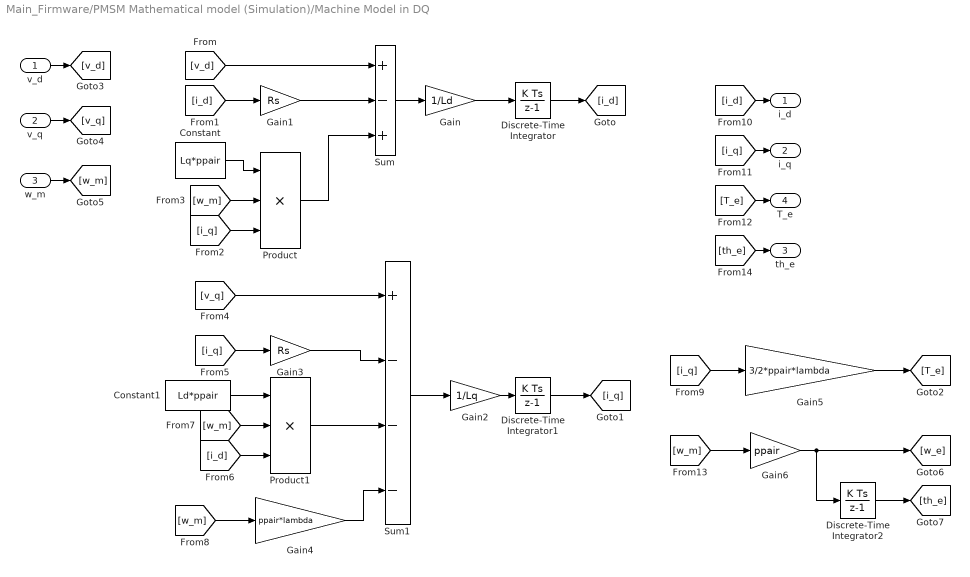
== system Main_Firmware/PMSM Mathematical model (Simulation)/Machine Model in DQ ==
  v_d : Inport
  v_q : Inport  Port=2
  w_m : Inport  Port=3
  Constant : Constant  Value=Lq*ppair
  Constant1 : Constant  Value=Ld*ppair
  Discrete-Time Integrator : DiscreteIntegrator  SampleTime=-1  ICPrevOutput=DiscIntNeverNeededParam  ICPrevScaledInput=DiscIntNeverNeededParam
  Discrete-Time Integrator1 : DiscreteIntegrator  SampleTime=-1  ICPrevOutput=DiscIntNeverNeededParam  ICPrevScaledInput=DiscIntNeverNeededParam
  Discrete-Time Integrator2 : DiscreteIntegrator  SampleTime=-1  ICPrevOutput=DiscIntNeverNeededParam  ICPrevScaledInput=DiscIntNeverNeededParam
  Gain : Gain  Gain=1/Ld
  Gain1 : Gain  Gain=Rs
  Gain2 : Gain  Gain=1/Lq
  Gain3 : Gain  Gain=Rs
  Gain4 : Gain  Gain=ppair*lambda
  Gain5 : Gain  Gain=3/2*ppair*lambda
  Gain6 : Gain  Gain=ppair
  Product : Product  Inputs=3
  Product1 : Product  Inputs=3
  Sum : Sum  Inputs=+-+
  Sum1 : Sum  Inputs=+---
  i_d : Outport
  i_q : Outport  Port=2
  th_e : Outport  Port=3
  T_e : Outport  Port=4
  wires:
  Constant/1 -> Product/1
  Product/1 -> Sum/3
  Discrete-Time Integrator/1 -> [i_d]
  [v_d] -> Sum/1
  [w_m] -> Product1/2
  Gain4/1 -> Sum1/4
  [i_q] -> Product/3
  Sum/1 -> Gain/1
  [w_m] -> Gain4/1
  [i_d] -> Gain1/1
  Sum1/1 -> Gain2/1
  Gain/1 -> Discrete-Time Integrator/1
  Gain5/1 -> [T_e]
  [i_q] -> Gain5/1
  Gain1/1 -> Sum/2
  Discrete-Time Integrator1/1 -> [i_q]
  [i_q] -> Gain3/1
  Product1/1 -> Sum1/3
  Constant1/1 -> Product1/1
  Gain2/1 -> Discrete-Time Integrator1/1
  [v_q] -> Sum1/1
  Gain3/1 -> Sum1/2
  [i_d] -> Product1/3
  [w_m] -> Product/2
  v_d/1 -> [v_d]
  v_q/1 -> [v_q]
  [i_d] -> i_d/1
  [i_q] -> i_q/1
  [T_e] -> T_e/1
  w_m/1 -> [w_m]
  [w_m] -> Gain6/1
  Gain6/1 -> Discrete-Time Integrator2/1, [w_e]
  Discrete-Time Integrator2/1 -> [th_e]
  [th_e] -> th_e/1

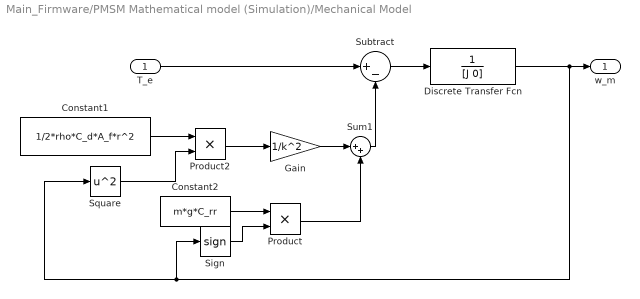
== system Main_Firmware/PMSM Mathematical model (Simulation)/Mechanical Model ==
  T_e : Inport
  Constant1 : Constant  Value=1/2*rho*C_d*A_f*r^2
  Constant2 : Constant  Value=m*g*C_rr
  Discrete Transfer Fcn : DiscreteTransferFcn  LoadFcn=dspblkCoreblockFVToolHelper(gcbh,'load');  Denominator=[J 0]
      settings: CopyFcn=dspblkCoreblockFVToolHelper(gcbh,'copy');  DeleteFcn=dspblkCoreblockFVToolHelper(gcbh,'close');  ModelCloseFcn=dspblkCoreblockFVToolHelper(gcbh,'close');  PreSaveFcn=dspblkCoreblockFVToolHelper(gcbh,'presave');  PostSaveFcn=dspblkCoreblockFVToolHelper(gcbh,'postsave');  CloseFcn=dspblkCoreblockFVToolHelper(gcbh,'close');
  Gain : Gain  Gain=1/k^2
  Product : Product
  Product2 : Product
  Sign : Signum
  Square : Math  Operator=square
  Subtract : Sum  Inputs=|+-
  Sum1 : Sum  Inputs=|++
  w_m : Outport
  wires:
  Constant1/1 -> Product2/1
  Discrete Transfer Fcn/1 -> Sign/1, Square/1, w_m/1
  Product2/1 -> Gain/1
  Square/1 -> Product2/2
  Subtract/1 -> Discrete Transfer Fcn/1
  T_e/1 -> Subtract/1
  Sum1/1 -> Subtract/2
  Gain/1 -> Sum1/1
  Constant2/1 -> Product/1
  Sign/1 -> Product/2
  Product/1 -> Sum1/2
